simulink model "complete_model_sim_nolib"  (R2023b)
settings: Solver=VariableStepAuto  StartTime=0.0  StopTime=1e4  RelTol=1e-3
values from neighbouring files (symbols this model uses):
  a = 6.851221970532768e+03    (= 6851.22197053)    [complete_model.m]
  alpha1 = 0.4    [complete_model.m]
  alpha2 = 0.1    [complete_model.m]
  alpha3 = 0.5    [complete_model.m]
  D = zeros(3)    [complete_model.m]
  e = 0    [complete_model.m]
  FOV_earth = deg2rad(33)    [complete_model.m]
  FOV_sun = deg2rad(100)    [complete_model.m]
  freq_earth = 5    [complete_model.m]
  freq_mag = 5    [complete_model.m]
  freq_sun = 5    [complete_model.m]
  I = diag([I1 I2 I3])    [complete_model.m]    (also in compute_integral.m = I + (y(i + 1) + y(i) ) * (t(i + 1) - t(i)) * 0.5)
  Iinv = I\eye(3)    [complete_model.m]
  jb = [0.01; 0.05; 0.01]    [complete_model.m]
  k_gain = (4*pi/T) * (1 + sin(chsi)) * I2    [complete_model.m]
  mu = astroConstants(13)    [complete_model.m]
  n = sqrt(mu/a^3)    [complete_model.m]
  omega0 = 0.06 * rand(3,1)    [complete_model.m]
  omegaE = deg2rad(15)/3600    [complete_model.m]
  rs = -rr    [complete_model.m]
  s0 = 2*pi*rand(3,1)    [complete_model.m]
  tol = 0.2    [complete_model.m]
undefined symbols (not defined in the file or in its folder): gh, magnitude
libraries: cstextras x3, matrix_library x2, simulink_extras x1
(part 2 of 3)

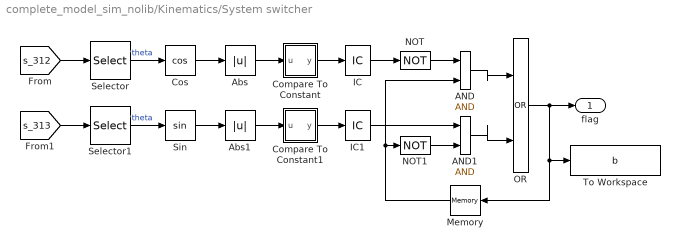
== system complete_model_sim_nolib/Kinematics/System switcher ==
  AND : Logic  IconShape=distinctive  AllPortsSameDT=off  OutDataTypeStr=boolean
  AND1 : Logic  IconShape=distinctive  AllPortsSameDT=off  OutDataTypeStr=boolean
  Abs : Abs  SaturateOnIntegerOverflow=off
  Abs1 : Abs  SaturateOnIntegerOverflow=off
  Compare To Constant : Subsystem  mask(Compare To Constant){relop=<, const=tol, OutDataTypeStr=boolean, ZeroCross=on}
      mask prompts: relop "Simulink:masks:Operator_MP"; const "Simulink:masks:ConstantValue_MP"; OutDataTypeStr "Simulink:masks:OutputDataType_MP"; ZeroCross "Simulink:masks:EnableZerocrossingDetection_MP"
      mask help: Simulink:masks:CompareToConstant_MD
      mask init: same as complete_model_sim_nolib/Control/De-Tumbling Bdot control1/Compare To Constant
      settings: LibrarySourceBlock=|
      | simulink/Logic and Bit
      | Operations/Compare
      | To Constant
      mask TypeOptions relop: == | ~= | < | <= | >= | >
      mask TypeOptions OutDataTypeStr: Simulink:masks:uint8 | Simulink:masks:boolean
      mask Callback ZeroCross: sl('zeroCrossEnable', gcbh);
      mask Display: disp(str)
  Compare To Constant1 : Subsystem  mask(Compare To Constant){relop=<, const=tol, OutDataTypeStr=boolean, ZeroCross=on}
      mask prompts: relop "Simulink:masks:Operator_MP"; const "Simulink:masks:ConstantValue_MP"; OutDataTypeStr "Simulink:masks:OutputDataType_MP"; ZeroCross "Simulink:masks:EnableZerocrossingDetection_MP"
      mask help: Simulink:masks:CompareToConstant_MD
      mask init: same as complete_model_sim_nolib/Control/De-Tumbling Bdot control1/Compare To Constant
      settings: LibrarySourceBlock=|
      | simulink/Logic and Bit
      | Operations/Compare
      | To Constant
      mask TypeOptions relop: == | ~= | < | <= | >= | >
      mask TypeOptions OutDataTypeStr: Simulink:masks:uint8 | Simulink:masks:boolean
      mask Callback ZeroCross: sl('zeroCrossEnable', gcbh);
      mask Display: disp(str)
  Cos : Trigonometry  Operator=cos
  IC : InitialCondition  Value=0
  IC1 : InitialCondition  Value=0
  Memory : Memory  InitialCondition=1
  NOT : Logic  Operator=NOT  IconShape=distinctive  AllPortsSameDT=off  OutDataTypeStr=boolean
  NOT1 : Logic  Operator=NOT  IconShape=distinctive  AllPortsSameDT=off  OutDataTypeStr=boolean
  OR : Logic  Operator=OR  IconShape=distinctive  AllPortsSameDT=off  OutDataTypeStr=boolean
  Selector : Selector  InputPortWidth=3  IndexOptions=Index vector (dialog)  Indices=2  OutputSizes=1
  Selector1 : Selector  InputPortWidth=3  IndexOptions=Index vector (dialog)  Indices=2  OutputSizes=1
  Sin : Trigonometry
  To Workspace : ToWorkspace  VariableName=b  SaveFormat=Timeseries  SampleTime=-1
  flag : Outport
  wires:
  Cos/1 -> Abs/1
  [s_312] -> Selector/1
  Compare To Constant/1(y) -> IC/1
  Selector1/1 -> Sin/1  "theta"
  Abs/1 -> Compare To Constant/1(u)
  Compare To Constant1/1(y) -> IC1/1
  Selector/1 -> Cos/1  "theta"
  Abs1/1 -> Compare To Constant1/1(u)
  Sin/1 -> Abs1/1
  [s_313] -> Selector1/1
  IC/1 -> NOT/1
  NOT/1 -> AND/1
  AND/1 -> OR/1
  NOT1/1 -> AND1/2
  IC1/1 -> AND1/1
  AND1/1 -> OR/2
  OR/1 -> To Workspace/1, Memory/1, flag/1
  Memory/1 -> AND/2, NOT1/1

== system complete_model_sim_nolib/Magnetometer/Band-Limited White Noise ==
  Output : Gain  Gain=sqrt(Cov)/sqrt(Ts(1))  SaturateOnIntegerOverflow=on  OutDataTypeStr=Inherit: Same as input  ParamDataTypeStr=Inherit: Same as input
  White Noise : RandomNumber  DisableCoverage=on  Seed=seed  SampleTime=Ts
  y : Outport
  wires:
  Output/1 -> y/1
  White Noise/1 -> Output/1

== system complete_model_sim_nolib/Magnetometer/Band-Limited White Noise1 ==
  Output : Gain  Gain=sqrt(Cov)/sqrt(Ts(1))  SaturateOnIntegerOverflow=on  OutDataTypeStr=Inherit: Same as input  ParamDataTypeStr=Inherit: Same as input
  White Noise : RandomNumber  DisableCoverage=on  Seed=seed  SampleTime=Ts
  y : Outport
  wires:
  Output/1 -> y/1
  White Noise/1 -> Output/1

== system complete_model_sim_nolib/Magnetometer/Band-Limited White Noise2 ==
  Output : Gain  Gain=sqrt(Cov)/sqrt(Ts(1))  SaturateOnIntegerOverflow=on  OutDataTypeStr=Inherit: Same as input  ParamDataTypeStr=Inherit: Same as input
  White Noise : RandomNumber  DisableCoverage=on  Seed=seed  SampleTime=Ts
  y : Outport
  wires:
  Output/1 -> y/1
  White Noise/1 -> Output/1

== system complete_model_sim_nolib/Magnetometer/Normalize Vector ==
  In1 : Inport
  Constant : Constant
  Demux : Demux  Outputs=[-1 1]
  Divide : Product  Inputs=*/  OutDataTypeStr=double
  Ground : Ground
  Math Function : Math  Operator=square  SignedPower=on
  Math Function1 : Math  Operator=sqrt  SignedPower=on
  Mux : Mux  Inputs=2
  Mux1 : Mux  Inputs=2
  Product : Product  RndMeth=Zero
  Sum of Elements : Sum  Inputs=+
  Switch : Switch  Criteria=u2 > Threshold  Threshold=maxzero  SaturateOnIntegerOverflow=off  InputSameDT=off
  Out1 : Outport  VectorParamsAs1DForOutWhenUnconnected=off
  wires:
  Ground/1 -> Product/2
  Product/1 -> Mux1/1
  Constant/1 -> Mux1/2
  Mux1/1 -> Switch/3
  Sum of Elements/1 -> Math Function1/1
  Math Function/1 -> Sum of Elements/1
  Demux/2 -> Divide/2
  Demux/1 -> Divide/1
  Switch/1 -> Demux/1
  Mux/1 -> Switch/1
  Math Function1/1 -> Mux/2, Switch/2
  In1/1 -> Product/1, Math Function/1, Mux/1
  Divide/1 -> Out1/1

== system complete_model_sim_nolib/Sun Sensor/FOV CHECK ==
  In1 : Inport
  Acos : Trigonometry  Operator=acos
  Dot Product : DotProduct  OutDataTypeStr=Inherit: Inherit via internal rule
  FOV angle : Constant  Value=FOV_sun
  Less Than : RelationalOperator  Operator=<  OutDataTypeStr=boolean  RndMeth=Simplest  InputSameDT=off
  optical axis : Constant  Value=[0;0;1]
  b : Outport
  wires:
  optical axis/1 -> Dot Product/1
  In1/1 -> Dot Product/2
  Dot Product/1 -> Acos/1
  FOV angle/1 -> Less Than/2
  Acos/1 -> Less Than/1
  Less Than/1 -> b/1

== system complete_model_sim_nolib/Sun Sensor/Sun Sensor Modeling ==
  Sb : Inport
  Cross Product : Subsystem  mask(CrossProduct){}
      mask help: Simulink:masks:MatLibCrossProduct_MD
      settings: LibrarySourceBlock=|
      | simulink/Matrix
      | Operations/Cross Product
      mask Display: disp('cross')
  Normalize Vector : Subsystem  mask(Normalize Vector){maxzero=0}
      mask prompts: maxzero "Maximum modulus to treat vector as zero:"
      mask help:
      | Normalize a vector.
      | Output is the unit vector parallel to the input vector. Input can be vector of any size.
      | If the modulus of the input is lower or equal than specified, the output is set to zeros(size(u)).
      settings: LibrarySourceBlock=vrlib/Utilities/Normalize Vector
      mask Help: helpview(vrmfunc('FnHelpTopic'), 'vr_normalizevector');
      mask Display: disp('Normalize')
  Normalize Vector1 : Subsystem  mask(Normalize Vector){maxzero=0}
      mask prompts: maxzero "Maximum modulus to treat vector as zero:"
      mask help:
      | Normalize a vector.
      | Output is the unit vector parallel to the input vector. Input can be vector of any size.
      | If the modulus of the input is lower or equal than specified, the output is set to zeros(size(u)).
      settings: LibrarySourceBlock=vrlib/Utilities/Normalize Vector
      mask Help: helpview(vrmfunc('FnHelpTopic'), 'vr_normalizevector');
      mask Display: disp('Normalize')
  Product : Product
  Random Number : RandomNumber  Variance=tan(deg2rad(1/60))^2*0.1  SampleTime=0.1
  Sum2 : Sum
  Uniform Random Number : UniformRandomNumber  SampleTime=1/freq_sun
  Uniform Random Number1 : UniformRandomNumber  SampleTime=1/freq_sun
  Uniform Random Number2 : UniformRandomNumber  SampleTime=1/freq_sun
  Vector Concatenate : Concatenate  NumInputs=3
  Zero-Order Hold : ZeroOrderHold  SampleTime=1/freq_sun
  s3 : Outport
  wires:
  Zero-Order Hold/1 -> Cross Product/2(b), Sum2/2  "Sb"
  Sum2/1 -> Normalize Vector/1(In1)  "q"
  Uniform Random Number1/1 -> Vector Concatenate/2
  Vector Concatenate/1 -> Cross Product/1(a)
  Uniform Random Number2/1 -> Vector Concatenate/3
  Normalize Vector/1(Out1) -> s3/1
  Uniform Random Number/1 -> Vector Concatenate/1
  Product/1 -> Sum2/1
  Random Number/1 -> Product/1
  Sb/1 -> Zero-Order Hold/1
  Cross Product/1(y) -> Normalize Vector1/1(In1)
  Normalize Vector1/1(Out1) -> Product/2

== system complete_model_sim_nolib/kep_dyn/r_norm ==
  e : Inport
  theta : Inport  Port=2
  Constant : Constant  Value=a
  Constant1 : Constant
  Cos : Trigonometry  Operator=cos
  Divide : Product  Inputs=*/
  Power : Math  Operator=magnitude^2
  Product : Product
  Product1 : Product
  Sum : Sum  Inputs=+-
  Sum2 : Sum
  r : Outport
  wires:
  e/1 -> Product1/2, Power/1
  Power/1 -> Sum/2
  Constant1/1 -> Sum2/2, Sum/1
  Sum/1 -> Product/2
  Constant/1 -> Product/1
  theta/1 -> Cos/1
  Cos/1 -> Product1/1
  Product1/1 -> Sum2/1
  Product/1 -> Divide/1
  Sum2/1 -> Divide/2
  Divide/1 -> r/1

== system complete_model_sim_nolib/kep_dyn/theta integration ==
  theta : Inport
  e : Inport  Port=2
  Constant : Constant  Value=n
  Constant2 : Constant
  Constant3 : Constant  Value=3/2
  Cos : Trigonometry  Operator=cos
  Divide : Product  Inputs=*/
  Math Function : Math  Operator=square
  Math Function1 : Math  Operator=square
  Math Function2 : Math  Operator=pow
  Product : Product
  Product1 : Product
  Sum : Sum
  Sum1 : Sum  Inputs=+-
  theta_dot : Outport
  wires:
  Product1/1 -> Divide/1
  Product/1 -> Sum/2
  Math Function2/1 -> Divide/2
  Sum1/1 -> Math Function2/1
  Constant2/1 -> Sum1/1, Sum/1
  Math Function1/1 -> Sum1/2
  e/1 -> Product/2, Math Function1/1
  Constant3/1 -> Math Function2/2
  Constant/1 -> Product1/1
  Sum/1 -> Math Function/1
  Math Function/1 -> Product1/2
  Cos/1 -> Product/1
  theta/1 -> Cos/1
  Divide/1 -> theta_dot/1

== system complete_model_sim_nolib/relative kinematics/Subsystem ==
  theta : Inport
  Constant3 : Constant
  Constant4 : Constant  Value=0
  Cos2 : Trigonometry  Operator=cos
  Cos3 : Trigonometry
  Gain : Gain  Gain=-1
  Matrix Concatenate1 : Concatenate  NumInputs=3  Mode=Multidimensional array  ConcatenateDimension=2
  Vector Concatenate : Concatenate  NumInputs=3
  Vector Concatenate1 : Concatenate  NumInputs=3
  Vector Concatenate2 : Concatenate  NumInputs=3
  A_PL : Outport
  wires:
  Constant4/1 -> Vector Concatenate2/2, Vector Concatenate/3, Vector Concatenate1/3, Vector Concatenate2/1
  Vector Concatenate/1 -> Matrix Concatenate1/1
  Cos2/1 -> Vector Concatenate1/2, Vector Concatenate/1
  Gain/1 -> Vector Concatenate1/1
  Cos3/1 -> Vector Concatenate/2, Gain/1
  Constant3/1 -> Vector Concatenate2/3
  Vector Concatenate2/1 -> Matrix Concatenate1/3
  Vector Concatenate1/1 -> Matrix Concatenate1/2
  theta/1 -> Cos2/1, Cos3/1
  Matrix Concatenate1/1 -> A_PL/1  "A_PL"

== system complete_model_sim_nolib/Attitude Determination  1/Enabled Subsystem/S ==
  q : Inport
  p : Inport  Port=2
  Cross Product : Subsystem  mask(CrossProduct){}
      mask help: Simulink:masks:MatLibCrossProduct_MD
      settings: LibrarySourceBlock=|
      | simulink/Matrix
      | Operations/Cross Product
      mask Display: disp('cross')
  Cross Product1 : Subsystem  mask(CrossProduct){}
      mask help: Simulink:masks:MatLibCrossProduct_MD
      settings: LibrarySourceBlock=|
      | simulink/Matrix
      | Operations/Cross Product
      mask Display: disp('cross')
  Matrix Concatenate : Concatenate  NumInputs=3  Mode=Multidimensional array  ConcatenateDimension=2
  Normalize Vector : Subsystem  mask(Normalize Vector){maxzero=0}
      mask prompts: maxzero "Maximum modulus to treat vector as zero:"
      mask help:
      | Normalize a vector.
      | Output is the unit vector parallel to the input vector. Input can be vector of any size.
      | If the modulus of the input is lower or equal than specified, the output is set to zeros(size(u)).
      settings: LibrarySourceBlock=vrlib/Utilities/Normalize Vector
      mask Help: helpview(vrmfunc('FnHelpTopic'), 'vr_normalizevector');
      mask Display: disp('Normalize')
  S : Outport
  wires:
  p/1 -> Matrix Concatenate/1, Cross Product/1(a), Cross Product1/1(a)
  q/1 -> Cross Product/2(b)
  Normalize Vector/1(Out1) -> Matrix Concatenate/2, Cross Product1/2(b)
  Matrix Concatenate/1 -> S/1
  Cross Product1/1(y) -> Matrix Concatenate/3
  Cross Product/1(y) -> Normalize Vector/1(In1)

== system complete_model_sim_nolib/Attitude Determination  1/Enabled Subsystem/V ==
  b : Inport
  a : Inport  Port=2
  Cross Product : Subsystem  mask(CrossProduct){}
      mask help: Simulink:masks:MatLibCrossProduct_MD
      settings: LibrarySourceBlock=|
      | simulink/Matrix
      | Operations/Cross Product
      mask Display: disp('cross')
  Cross Product1 : Subsystem  mask(CrossProduct){}
      mask help: Simulink:masks:MatLibCrossProduct_MD
      settings: LibrarySourceBlock=|
      | simulink/Matrix
      | Operations/Cross Product
      mask Display: disp('cross')
  Matrix Concatenate : Concatenate  NumInputs=3  Mode=Multidimensional array  ConcatenateDimension=2
  Normalize Vector : Subsystem  mask(Normalize Vector){maxzero=0}
      mask prompts: maxzero "Maximum modulus to treat vector as zero:"
      mask help:
      | Normalize a vector.
      | Output is the unit vector parallel to the input vector. Input can be vector of any size.
      | If the modulus of the input is lower or equal than specified, the output is set to zeros(size(u)).
      settings: LibrarySourceBlock=vrlib/Utilities/Normalize Vector
      mask Help: helpview(vrmfunc('FnHelpTopic'), 'vr_normalizevector');
      mask Display: disp('Normalize')
  V : Outport
  wires:
  Cross Product1/1(y) -> Matrix Concatenate/3
  Matrix Concatenate/1 -> V/1
  Normalize Vector/1(Out1) -> Cross Product1/2(b), Matrix Concatenate/2
  Cross Product/1(y) -> Normalize Vector/1(In1)
  b/1 -> Cross Product/2(b)
  a/1 -> Cross Product1/1(a), Cross Product/1(a), Matrix Concatenate/1

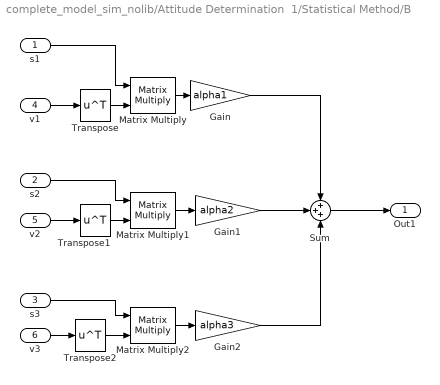
== system complete_model_sim_nolib/Attitude Determination  1/Statistical Method/B ==
  s1 : Inport
  s2 : Inport  Port=2
  s3 : Inport  Port=3
  v1 : Inport  Port=4
  v2 : Inport  Port=5
  v3 : Inport  Port=6
  Gain : Gain  Gain=alpha1
  Gain1 : Gain  Gain=alpha2
  Gain2 : Gain  Gain=alpha3
  Matrix Multiply : Product  Multiplication=Matrix(*)
  Matrix Multiply1 : Product  Multiplication=Matrix(*)
  Matrix Multiply2 : Product  Multiplication=Matrix(*)
  Sum : Sum  Inputs=+++
  Transpose : Math  Operator=transpose
  Transpose1 : Math  Operator=transpose
  Transpose2 : Math  Operator=transpose
  Out1 : Outport
  wires:
  v1/1 -> Transpose/1
  Transpose/1 -> Matrix Multiply/2
  s1/1 -> Matrix Multiply/1
  Transpose1/1 -> Matrix Multiply1/2
  s2/1 -> Matrix Multiply1/1
  Transpose2/1 -> Matrix Multiply2/2
  v3/1 -> Transpose2/1
  Sum/1 -> Out1/1
  Matrix Multiply/1 -> Gain/1
  Matrix Multiply1/1 -> Gain1/1
  Matrix Multiply2/1 -> Gain2/1
  Gain/1 -> Sum/1
  Gain1/1 -> Sum/2
  Gain2/1 -> Sum/3
  v2/1 -> Transpose1/1
  s3/1 -> Matrix Multiply2/1

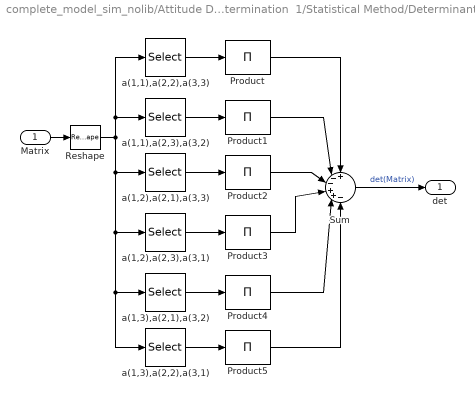
== system complete_model_sim_nolib/Attitude Determination  1/Statistical Method/Determinant of 3x3 Matrix ==
  Matrix : Inport  PortDimensions=[3 3]
  Product{,1..5} (6 alike) : Product  Inputs=1  SaturateOnIntegerOverflow=on  OutDataTypeStr=Inherit: Same as first input
  Reshape : Reshape  OutputDimensionality=Column vector (2-D)
  Sum : Sum  Inputs=+--++-  SaturateOnIntegerOverflow=on
  a(1,1),a(2,2),a(3,3) : Selector  InputPortWidth=9  IndexOptions=Index vector (dialog)  Indices=[1 5 9]  OutputSizes=1
  a(1,1),a(2,3),a(3,2) : Selector  InputPortWidth=9  IndexOptions=Index vector (dialog)  Indices=[1 6 8]  OutputSizes=1
  a(1,2),a(2,1),a(3,3) : Selector  InputPortWidth=9  IndexOptions=Index vector (dialog)  Indices=[2 4 9]  OutputSizes=1
  a(1,2),a(2,3),a(3,1) : Selector  InputPortWidth=9  IndexOptions=Index vector (dialog)  Indices=[3 4 8]  OutputSizes=1
  a(1,3),a(2,1),a(3,2) : Selector  InputPortWidth=9  IndexOptions=Index vector (dialog)  Indices=[2 6 7]  OutputSizes=1
  a(1,3),a(2,2),a(3,1) : Selector  InputPortWidth=9  IndexOptions=Index vector (dialog)  Indices=[3 5 7]  OutputSizes=1
  det : Outport  PortDimensions=1  VectorParamsAs1DForOutWhenUnconnected=off
  wires:
  Reshape/1 -> a(1,1),a(2,3),a(3,2)/1, a(1,1),a(2,2),a(3,3)/1, a(1,3),a(2,2),a(3,1)/1, a(1,3),a(2,1),a(3,2)/1, a(1,2),a(2,3),a(3,1)/1, a(1,2),a(2,1),a(3,3)/1
  Sum/1 -> det/1  "det(Matrix)"
  Matrix/1 -> Reshape/1
  Product5/1 -> Sum/6
  Product4/1 -> Sum/5
  Product3/1 -> Sum/4
  Product2/1 -> Sum/3
  Product1/1 -> Sum/2
  Product/1 -> Sum/1
  a(1,3),a(2,2),a(3,1)/1 -> Product5/1
  a(1,3),a(2,1),a(3,2)/1 -> Product4/1
  a(1,2),a(2,3),a(3,1)/1 -> Product3/1
  a(1,2),a(2,1),a(3,3)/1 -> Product2/1
  a(1,1),a(2,3),a(3,2)/1 -> Product1/1
  a(1,1),a(2,2),a(3,3)/1 -> Product/1

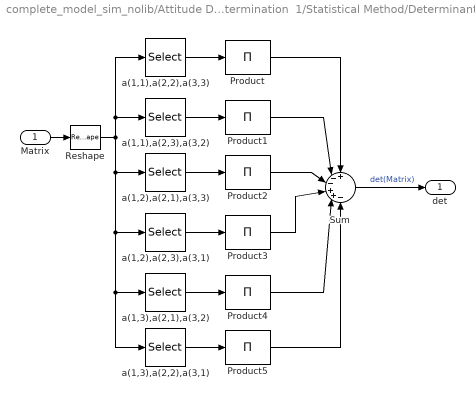
== system complete_model_sim_nolib/Attitude Determination  1/Statistical Method/Determinant of 3x3 Matrix1 ==
  Matrix : Inport  PortDimensions=[3 3]
  Product{,1..5} (6 alike) : Product  Inputs=1  SaturateOnIntegerOverflow=on  OutDataTypeStr=Inherit: Same as first input
  Reshape : Reshape  OutputDimensionality=Column vector (2-D)
  Sum : Sum  Inputs=+--++-  SaturateOnIntegerOverflow=on
  a(1,1),a(2,2),a(3,3) : Selector  InputPortWidth=9  IndexOptions=Index vector (dialog)  Indices=[1 5 9]  OutputSizes=1
  a(1,1),a(2,3),a(3,2) : Selector  InputPortWidth=9  IndexOptions=Index vector (dialog)  Indices=[1 6 8]  OutputSizes=1
  a(1,2),a(2,1),a(3,3) : Selector  InputPortWidth=9  IndexOptions=Index vector (dialog)  Indices=[2 4 9]  OutputSizes=1
  a(1,2),a(2,3),a(3,1) : Selector  InputPortWidth=9  IndexOptions=Index vector (dialog)  Indices=[3 4 8]  OutputSizes=1
  a(1,3),a(2,1),a(3,2) : Selector  InputPortWidth=9  IndexOptions=Index vector (dialog)  Indices=[2 6 7]  OutputSizes=1
  a(1,3),a(2,2),a(3,1) : Selector  InputPortWidth=9  IndexOptions=Index vector (dialog)  Indices=[3 5 7]  OutputSizes=1
  det : Outport  PortDimensions=1  VectorParamsAs1DForOutWhenUnconnected=off
  wires:
  a(1,1),a(2,2),a(3,3)/1 -> Product/1
  a(1,1),a(2,3),a(3,2)/1 -> Product1/1
  a(1,2),a(2,1),a(3,3)/1 -> Product2/1
  a(1,2),a(2,3),a(3,1)/1 -> Product3/1
  a(1,3),a(2,1),a(3,2)/1 -> Product4/1
  a(1,3),a(2,2),a(3,1)/1 -> Product5/1
  Product/1 -> Sum/1
  Product1/1 -> Sum/2
  Product2/1 -> Sum/3
  Product3/1 -> Sum/4
  Product4/1 -> Sum/5
  Product5/1 -> Sum/6
  Matrix/1 -> Reshape/1
  Sum/1 -> det/1  "det(Matrix)"
  Reshape/1 -> a(1,2),a(2,1),a(3,3)/1, a(1,2),a(2,3),a(3,1)/1, a(1,3),a(2,1),a(3,2)/1, a(1,3),a(2,2),a(3,1)/1, a(1,1),a(2,2),a(3,3)/1, a(1,1),a(2,3),a(3,2)/1

== system complete_model_sim_nolib/Control/De-Tumbling Bdot control1/Compare To Constant ==
  u : Inport
  Compare : RelationalOperator  OutDataTypeStr=boolean
  Constant : Constant  DisableCoverage=on  Value=const  OutDataTypeStr=Inherit: Inherit via back propagation
  y : Outport
  wires:
  u/1 -> Compare/1
  Constant/1 -> Compare/2
  Compare/1 -> y/1

== system complete_model_sim_nolib/Control/De-Tumbling Bdot control1/Compare To Constant1 ==
  u : Inport
  Compare : RelationalOperator  Operator=<=  OutDataTypeStr=boolean
  Constant : Constant  DisableCoverage=on  Value=const  OutDataTypeStr=Inherit: Inherit via back propagation
  y : Outport
  wires:
  u/1 -> Compare/1
  Constant/1 -> Compare/2
  Compare/1 -> y/1

== system complete_model_sim_nolib/Control/De-Tumbling Bdot control1/Discrete Derivative1 ==
  note: ( U(k) - U(k-1) )
  note: U(k)
  U : Inport
  Data Type Duplicate : DataTypeDuplicate  DisableCoverage=on  NumInputPorts=3
  Diff : Sum  Description=Add in CPU  Inputs=+-  OutMin=OutMin  OutMax=OutMax  OutDataTypeStr=diffDT
  TSamp : SampleTimeMath  DisableCoverage=on  TsampMathOp=/  weightValue=inverseGainval  TsampMathImp=Offline Scaling Adjustment
  UD : UnitDelay  Description=Store in Global RAM  DisableCoverage=on  InitialCondition=ICPrevScaledInput  SampleTime=-1  HasFrameUpgradeWarning=on
  Y : Outport  OutMin=OutMin  OutMax=OutMax  InitialOutput=0
  wires:
  U/1 -> TSamp/1
  UD/1 -> Diff/2, Data Type Duplicate/3  "U(k-1)"
  Diff/1 -> Y/1, Data Type Duplicate/1
  TSamp/1 -> UD/1, Diff/1, Data Type Duplicate/2

== system complete_model_sim_nolib/Control/De-Tumbling Bdot control1/Discrete Varying Lowpass1 ==
  u : Inport
  frequency : Inport  Port=2
  FOS : cstextras/DiscreteFirstOrderSection  VariantControl=(default)  Ts=Ts  w0=w0
  y : Outport  VectorParamsAs1DForOutWhenUnconnected=off
  wires:
  u/1 -> FOS/1
  frequency/1 -> FOS/2
  FOS/1 -> y/1

== system complete_model_sim_nolib/Control/De-Tumbling Bdot control1/Normalize Vector ==
  In1 : Inport
  Constant : Constant
  Demux : Demux  Outputs=[-1 1]
  Divide : Product  Inputs=*/  OutDataTypeStr=double
  Ground : Ground
  Math Function : Math  Operator=square  SignedPower=on
  Math Function1 : Math  Operator=sqrt  SignedPower=on
  Mux : Mux  Inputs=2
  Mux1 : Mux  Inputs=2
  Product : Product  RndMeth=Zero
  Sum of Elements : Sum  Inputs=+
  Switch : Switch  Criteria=u2 > Threshold  Threshold=maxzero  SaturateOnIntegerOverflow=off  InputSameDT=off
  Out1 : Outport  VectorParamsAs1DForOutWhenUnconnected=off
  wires:
  Ground/1 -> Product/2
  Product/1 -> Mux1/1
  Constant/1 -> Mux1/2
  Mux1/1 -> Switch/3
  Sum of Elements/1 -> Math Function1/1
  Math Function/1 -> Sum of Elements/1
  Demux/2 -> Divide/2
  Demux/1 -> Divide/1
  Switch/1 -> Demux/1
  Mux/1 -> Switch/1
  Math Function1/1 -> Mux/2, Switch/2
  In1/1 -> Product/1, Math Function/1, Mux/1
  Divide/1 -> Out1/1

== system complete_model_sim_nolib/Control/Slew Maneuver/Control Logic ==
  u : Inport
  B_m : Inport  Port=2
  Abs1 : Abs  SaturateOnIntegerOverflow=off
  Compare To Constant : Subsystem  mask(Compare To Constant){relop=>, const=1e-5, OutDataTypeStr=boolean, ZeroCross=on}
      mask prompts: relop "Simulink:masks:Operator_MP"; const "Simulink:masks:ConstantValue_MP"; OutDataTypeStr "Simulink:masks:OutputDataType_MP"; ZeroCross "Simulink:masks:EnableZerocrossingDetection_MP"
      mask help: Simulink:masks:CompareToConstant_MD
      mask init: same as complete_model_sim_nolib/Control/De-Tumbling Bdot control1/Compare To Constant
      settings: LibrarySourceBlock=|
      | simulink/Logic and Bit
      | Operations/Compare
      | To Constant
      mask TypeOptions relop: == | ~= | < | <= | >= | >
      mask TypeOptions OutDataTypeStr: Simulink:masks:uint8 | Simulink:masks:boolean
      mask Callback ZeroCross: sl('zeroCrossEnable', gcbh);
      mask Display: disp(str)
  Merge1 : Merge
  NOT : Logic  Operator=NOT  IconShape=distinctive  AllPortsSameDT=off  OutDataTypeStr=boolean
  Selector1 : Selector  InputPortWidth=3  IndexOptions=Index vector (dialog)  Indices=1  OutputSizes=1
  Subsystem : Subsystem
  Subsystem1 : Subsystem
  cmd : Outport
  wires:
  Abs1/1 -> Compare To Constant/1(u)
  Selector1/1 -> Abs1/1
  NOT/1 -> Subsystem/Enable
  Subsystem1/1(Out1) -> Merge1/1
  Compare To Constant/1(y) -> NOT/1, Subsystem1/Enable
  Subsystem/1(Out1) -> Merge1/2
  B_m/1 -> Selector1/1, Subsystem/1(Bm), Subsystem1/1(B_m)
  u/1 -> Subsystem/2(u), Subsystem1/2(u)
  Merge1/1 -> cmd/1

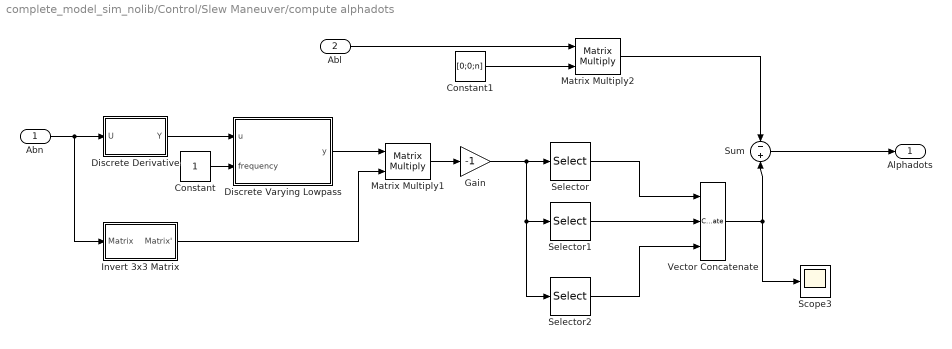
== system complete_model_sim_nolib/Control/Slew Maneuver/compute alphadots ==
  Abn : Inport
  Abl : Inport  Port=2
  Constant : Constant
  Constant1 : Constant  Value=[0;0;n]
  Discrete Derivative : Subsystem  mask(Discrete Derivative){gainval=1.0, ICPrevScaledInput=0.0, InputProcessing=Elements as channels (sample based), OutMin=[], OutMax=[], OutDataTypeStr=Inherit: Inherit via internal rule, OutputDataTypeScalingMode=Inherit via internal rule, OutDataType=fixdt(1, 16), OutScaling=2^-10, LockScale=off, RndMeth=Floor, DoSatur=off}
      mask prompts: gainval "Simulink:masks:GainValue_MP"; ICPrevScaledInput "Simulink:masks:InitialConditionForPreviousWeightedInputKuTs_MP"; InputProcessing "Simulink:masks:InputProcessing_MP"; OutMin "Simulink:masks:OutputMinimum_MP"; OutMax "Simulink:masks:OutputMaximum_MP"; OutDataTypeStr "Simulink:masks:OutputDataType_MP"; OutputDataTypeScalingMode "Simulink:masks:OutputDataTypeMode_MP"; OutDataType "Simulink:masks:OutputDataTypeegFixdt116Fixdtsingle_MP"; OutScaling "Simulink:masks:OutputScalingSlopeEg29OrSlopeBias_MP"; LockScale "Simulink:masks:LockOutputDataTypeAgainstFxpTools_MP"; RndMeth "Simulink:masks:IntegerRoundingMode_MP"; DoSatur "Simulink:masks:SaturateToMaxOrMinWhenOverflowsOccur_MP"
      mask help: Simulink:masks:DiscreteDerivative_MD
      mask init: same as complete_model_sim_nolib/Control/De-Tumbling Bdot control1/Discrete Derivative1
      settings: LibrarySourceBlock=simulink/Discrete/Discrete Derivative
      mask TypeOptions InputProcessing: Simulink:masks:ColumnsAsChannelsFrameBased | Simulink:masks:ElementsAsChannelsSampleBased
      mask Callback OutDataTypeStr: fixptdialog(gcbh)
      mask TypeOptions OutputDataTypeScalingMode: double | single | int8 | uint8 | int16 | uint16 | int32 | uint32 | Specify via dialog | Inherit via internal rule | Inherit via back propagation
      mask Callback OutputDataTypeScalingMode: fixptdialog(gcbh)
      mask Callback OutDataType: fixptdialog(gcbh)
      mask TypeOptions RndMeth: Simulink:masks:Ceiling | Simulink:masks:Convergent | Simulink:masks:Floor | Simulink:masks:Nearest | Simulink:masks:Round | Simulink:masks:Simplest | Simulink:masks:Zero
      mask Display: text(0.5, 0.5, 'K (z-1)', 'horizontalAlignment', 'center', 'verticalAlignment', 'bottom');text(0.5, 0.5, 'Ts z', 'horizontalAlignment', 'center', 'verticalAlignment', 'top');plot([0.3 0.7],[0.5 0.5]);
  Discrete Varying Lowpass : Subsystem  mask(Discrete Varying Lowpass){N=1, w0=0, Ts=1/30}
      mask prompts: N "Control:simulink:VaryingLowpassLabel1"; w0 "Control:simulink:VaryingLowpassLabel2"; Ts "Control:simulink:VaryingLowpassLabel3"
      mask help: Control:simulink:VaryingLowpass2
      mask init: same as complete_model_sim_nolib/ Actuators/Discrete Varying Lowpass
      settings: LibrarySourceBlock=cstblocks/Linear Parameter Varying/Discrete Varying Lowpass
      mask Help: eval('helpview(''control'',''VaryingLowpassDT'');')
      mask DialogControl N Prompt: Filter order:
      mask DialogControl w0 Prompt: Pre-warping frequency w0 (rad/s):
      mask DialogControl Ts Prompt: Sample time Ts:
      mask Display:
      | image('lowpass_dt.png',[0.1 0 0.8 1]);
      | port_label('input', 2, 'freq');
  Gain : Gain  Gain=-1
  Invert 3x3 Matrix : Subsystem
      settings: LibrarySourceBlock=|
      | aerolibutil/Invert
      | 3x3 Matrix
  Matrix Multiply1 : Product  Multiplication=Matrix(*)
  Matrix Multiply2 : Product  Multiplication=Matrix(*)
  Scope3 : Scope
  Selector : Selector  NumberOfDimensions=2  InputPortWidth=3  IndexOptions=Index vector (dialog),Index vector (dialog)  Indices=3,2  OutputSizes=1,1
  Selector1 : Selector  NumberOfDimensions=2  InputPortWidth=3  IndexOptions=Index vector (dialog),Index vector (dialog)  Indices=1,3  OutputSizes=1,1
  Selector2 : Selector  NumberOfDimensions=2  InputPortWidth=3  IndexOptions=Index vector (dialog),Index vector (dialog)  Indices=2,1  OutputSizes=1,1
  Sum : Sum  Inputs=-+
  Vector Concatenate : Concatenate  NumInputs=3
  Alphadots : Outport
  wires:
  Selector/1 -> Vector Concatenate/1
  Matrix Multiply2/1 -> Sum/1
  Discrete Varying Lowpass/1(y) -> Matrix Multiply1/1
  Matrix Multiply1/1 -> Gain/1
  Constant1/1 -> Matrix Multiply2/2
  Abn/1 -> Invert 3x3 Matrix/1(Matrix), Discrete Derivative/1(U)
  Invert 3x3 Matrix/1(Matrix') -> Matrix Multiply1/2
  Gain/1 -> Selector2/1, Selector1/1, Selector/1
  Constant/1 -> Discrete Varying Lowpass/2(frequency)
  Sum/1 -> Alphadots/1
  Selector2/1 -> Vector Concatenate/3
  Selector1/1 -> Vector Concatenate/2
  Discrete Derivative/1(Y) -> Discrete Varying Lowpass/1(u)
  Vector Concatenate/1 -> Sum/2, Scope3/1
  Abl/1 -> Matrix Multiply2/1

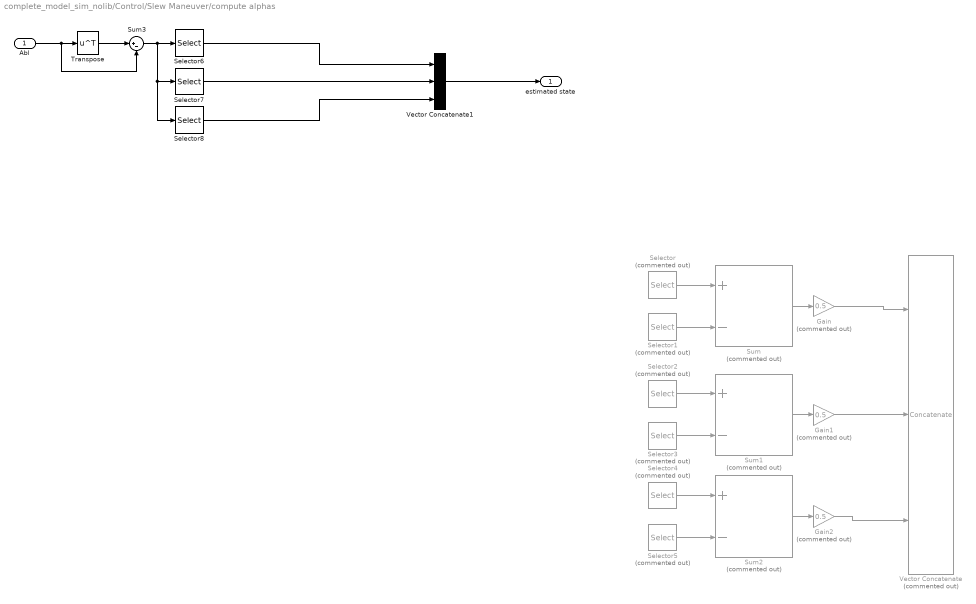
== system complete_model_sim_nolib/Control/Slew Maneuver/compute alphas ==
  Abl : Inport
  Gain : Gain  Commented=on  Gain=0.5
  Gain1 : Gain  Commented=on  Gain=0.5
  Gain2 : Gain  Commented=on  Gain=0.5
  Selector : Selector  Commented=on  NumberOfDimensions=2  InputPortWidth=3  IndexOptions=Index vector (dialog),Index vector (dialog)  Indices=2,3  OutputSizes=1,1
  Selector1 : Selector  Commented=on  NumberOfDimensions=2  InputPortWidth=3  IndexOptions=Index vector (dialog),Index vector (dialog)  Indices=3,2  OutputSizes=1,1
  Selector2 : Selector  Commented=on  NumberOfDimensions=2  InputPortWidth=3  IndexOptions=Index vector (dialog),Index vector (dialog)  Indices=3,1  OutputSizes=1,1
  Selector3 : Selector  Commented=on  NumberOfDimensions=2  InputPortWidth=3  IndexOptions=Index vector (dialog),Index vector (dialog)  Indices=1,3  OutputSizes=1,1
  Selector4 : Selector  Commented=on  NumberOfDimensions=2  InputPortWidth=3  IndexOptions=Index vector (dialog),Index vector (dialog)  Indices=1,2  OutputSizes=1,1
  Selector5 : Selector  Commented=on  NumberOfDimensions=2  InputPortWidth=3  IndexOptions=Index vector (dialog),Index vector (dialog)  Indices=2,1  OutputSizes=1,1
  Selector6 : Selector  NumberOfDimensions=2  InputPortWidth=3  IndexOptions=Index vector (dialog),Index vector (dialog)  Indices=3,2  OutputSizes=1,1
  Selector7 : Selector  NumberOfDimensions=2  InputPortWidth=3  IndexOptions=Index vector (dialog),Index vector (dialog)  Indices=1,3  OutputSizes=1,1
  Selector8 : Selector  NumberOfDimensions=2  InputPortWidth=3  IndexOptions=Index vector (dialog),Index vector (dialog)  Indices=2,1  OutputSizes=1,1
  Sum : Sum  Commented=on  Inputs=+-
  Sum1 : Sum  Commented=on  Inputs=+-
  Sum2 : Sum  Commented=on  Inputs=+-
  Sum3 : Sum  Inputs=|+-
  Transpose : Math  Operator=transpose
  Vector Concatenate : Concatenate  Commented=on  NumInputs=3
  Vector Concatenate1 : Concatenate  NumInputs=3
  estimated state : Outport
  wires:
  Selector1/1 -> Sum/2
  Selector/1 -> Sum/1
  Sum/1 -> Gain/1
  Selector2/1 -> Sum1/1
  Selector3/1 -> Sum1/2
  Selector4/1 -> Sum2/1
  Selector5/1 -> Sum2/2
  Sum1/1 -> Gain1/1
  Sum2/1 -> Gain2/1
  Gain/1 -> Vector Concatenate/1
  Gain1/1 -> Vector Concatenate/2
  Gain2/1 -> Vector Concatenate/3
  Abl/1 -> Sum3/2, Transpose/1
  Transpose/1 -> Sum3/1
  Sum3/1 -> Selector8/1, Selector7/1, Selector6/1
  Vector Concatenate1/1 -> estimated state/1
  Selector7/1 -> Vector Concatenate1/2
  Selector6/1 -> Vector Concatenate1/1
  Selector8/1 -> Vector Concatenate1/3

== system complete_model_sim_nolib/Disturbances/Magnetic Torque /compute Bn ==
  rN : Inport
  Cartesian to Spherical : simulink_extras/Transformations/Cartesian to Spherical
  Constant : Constant  Value=gh
  Demux : Demux  Outputs=3
  MATLAB Function : MATLAB Function  TreatAsAtomicUnit=on
  Matrix Multiply : Product  Multiplication=Matrix(*)
  Matrix Multiply1 : Product  Multiplication=Matrix(*)
  Subsystem : Subsystem
  Transpose : Math  Operator=transpose
  Bn : Outport
  wires:
  Subsystem/1(R_EN) -> Matrix Multiply/1, Transpose/1
  rN/1 -> Matrix Multiply/2
  Demux/1 -> Cartesian to Spherical/1
  Demux/2 -> Cartesian to Spherical/2
  Demux/3 -> Cartesian to Spherical/3
  Matrix Multiply/1 -> Demux/1
  Cartesian to Spherical/1 -> MATLAB Function/1(r)
  Cartesian to Spherical/2 -> MATLAB Function/2(theta)
  Cartesian to Spherical/3 -> MATLAB Function/3(phi)
  Transpose/1 -> Matrix Multiply1/1
  MATLAB Function/1(B) -> Matrix Multiply1/2
  Matrix Multiply1/1 -> Bn/1
  Constant/1 -> MATLAB Function/4(gh)

== system complete_model_sim_nolib/Horizon Sensor/EH sensor modeling/Cross Product ==
  note: Cross product of two 3x1 vectors a=[a1 a2 a3], b=[b1 b2 b3]:
      | y = a x b = (a2b3-a3b2)i + (a3b1-a1b3)j + (a1b2-a2b1)k
  a : Inport
  b : Inport  Port=2
  Element Product : Product  RndMeth=Simplest
  Selector2 : Selector  InputPortWidth=6  IndexOptions=Index vector (dialog)  Indices=[1 2 3]  OutputSizes=1
  Selector3 : Selector  InputPortWidth=6  IndexOptions=Index vector (dialog)  Indices=[4 5 6]  OutputSizes=1
  Sum : Sum  Inputs=+|-  RndMeth=Simplest
  a elements : Selector  InputPortWidth=3  IndexOptions=Index vector (dialog)  Indices=[2 3 1 3 1 2]  OutputSizes=1
  b elements : Selector  InputPortWidth=3  IndexOptions=Index vector (dialog)  Indices=[3 1 2 2 3 1]  OutputSizes=1
  y : Outport
  wires:
  Selector3/1 -> Sum/2
  Selector2/1 -> Sum/1
  Element Product/1 -> Selector2/1, Selector3/1
  b/1 -> b elements/1
  b elements/1 -> Element Product/2
  a elements/1 -> Element Product/1
  Sum/1 -> y/1
  a/1 -> a elements/1

== system complete_model_sim_nolib/Horizon Sensor/EH sensor modeling/Normalize Vector ==
  In1 : Inport
  Constant : Constant
  Demux : Demux  Outputs=[-1 1]
  Divide : Product  Inputs=*/  OutDataTypeStr=double
  Ground : Ground
  Math Function : Math  Operator=square  SignedPower=on
  Math Function1 : Math  Operator=sqrt  SignedPower=on
  Mux : Mux  Inputs=2
  Mux1 : Mux  Inputs=2
  Product : Product  RndMeth=Zero
  Sum of Elements : Sum  Inputs=+
  Switch : Switch  Criteria=u2 > Threshold  Threshold=maxzero  SaturateOnIntegerOverflow=off  InputSameDT=off
  Out1 : Outport  VectorParamsAs1DForOutWhenUnconnected=off
  wires:
  Ground/1 -> Product/2
  Product/1 -> Mux1/1
  Constant/1 -> Mux1/2
  Mux1/1 -> Switch/3
  Sum of Elements/1 -> Math Function1/1
  Math Function/1 -> Sum of Elements/1
  Demux/2 -> Divide/2
  Demux/1 -> Divide/1
  Switch/1 -> Demux/1
  Mux/1 -> Switch/1
  Math Function1/1 -> Mux/2, Switch/2
  In1/1 -> Product/1, Math Function/1, Mux/1
  Divide/1 -> Out1/1

== system complete_model_sim_nolib/Kinematics/Kinematics 312/A - s_312 ==
  A : Inport
  Asin : Trigonometry  Operator=asin
  Atan1 : Trigonometry  Operator=atan2
  Atan2 : Trigonometry  Operator=atan2
  Gain : Gain  Gain=-1
  Gain1 : Gain  Gain=-1
  Mux : Mux  Inputs=3
  Selector : Selector  NumberOfDimensions=2  InputPortWidth=3  IndexOptions=Index vector (dialog),Index vector (dialog)  Indices=2,1  OutputSizes=1,1
  Selector1 : Selector  NumberOfDimensions=2  InputPortWidth=3  IndexOptions=Index vector (dialog),Index vector (dialog)  Indices=2,2  OutputSizes=1,1
  Selector2 : Selector  NumberOfDimensions=2  InputPortWidth=3  IndexOptions=Index vector (dialog),Index vector (dialog)  Indices=2,3  OutputSizes=1,1
  Selector3 : Selector  NumberOfDimensions=2  InputPortWidth=3  IndexOptions=Index vector (dialog),Index vector (dialog)  Indices=1,3  OutputSizes=1,1
  Selector4 : Selector  NumberOfDimensions=2  InputPortWidth=3  IndexOptions=Index vector (dialog),Index vector (dialog)  Indices=3,3  OutputSizes=1,1
  s : Outport
  wires:
  Mux/1 -> s/1
  Selector4/1 -> Atan1/2  "a33"
  Atan1/1 -> Mux/3  "psi"
  Atan2/1 -> Mux/1  "phi"
  A/1 -> Selector2/1, Selector1/1, Selector/1, Selector3/1, Selector4/1
  Selector2/1 -> Asin/1  "a23"
  Selector3/1 -> Gain1/1  "a13"
  Selector1/1 -> Atan2/2  "a22"
  Selector/1 -> Gain/1  "a21"
  Asin/1 -> Mux/2  "theta"
  Gain/1 -> Atan2/1
  Gain1/1 -> Atan1/1

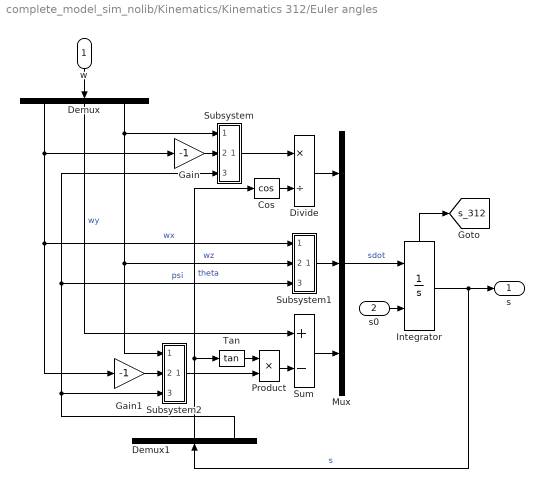
== system complete_model_sim_nolib/Kinematics/Kinematics 312/Euler angles ==
  w : Inport
  s0 : Inport  Port=2
  Cos : Trigonometry  Operator=cos
  Demux : Demux  Outputs=3
  Demux1 : Demux  Outputs=3
  Divide : Product  Inputs=*/
  Gain : Gain  Gain=-1
  Gain1 : Gain  Gain=-1
  Integrator : Integrator  InitialConditionSource=external  InitialCondition=s0  WrapState=on  WrappedStateUpperValue=2*pi  WrappedStateLowerValue=0  ShowStatePort=on
  Mux : Mux  Inputs=3
  Product : Product
  Subsystem : Subsystem
  Subsystem1 : Subsystem
  Subsystem2 : Subsystem
  Sum : Sum  Inputs=+-
  Tan : Trigonometry  Operator=tan
  s : Outport
  tag scope: s_312=global
  wires:
  w/1 -> Demux/1
  Integrator/1 -> Demux1/1, s/1  "s"
  Demux/3 -> Subsystem2/1(In1), Subsystem1/2(In2), Subsystem/1(In1)  "wz"
  Gain/1 -> Subsystem/2(In2)
  Demux/1 -> Gain1/1, Subsystem1/1(In1), Gain/1  "wx"
  Demux1/3 -> Subsystem2/3(In3), Subsystem1/3(In3), Subsystem/3(In3)  "psi"
  Subsystem/1(Out1) -> Divide/1
  Cos/1 -> Divide/2
  Demux1/2 -> Cos/1, Tan/1  "theta"
  Divide/1 -> Mux/1
  Subsystem1/1(Out1) -> Mux/2
  Gain1/1 -> Subsystem2/2(In2)
  Tan/1 -> Product/1
  Subsystem2/1(Out1) -> Product/2
  Product/1 -> Sum/2
  Demux/2 -> Sum/1  "wy"
  Sum/1 -> Mux/3
  Mux/1 -> Integrator/1  "sdot"
  s0/1 -> Integrator/2
  Integrator/State -> [s_312]

== system complete_model_sim_nolib/Kinematics/Kinematics 312/s_312 - A ==
  s : Inport
  Demux : Demux  Outputs=3
  Product : Product  Inputs=3  Multiplication=Matrix(*)
  R1 : Subsystem
  R2 : Subsystem
  R3 : Subsystem
  A : Outport
  wires:
  s/1 -> Demux/1  "s"
  R1/1(R1) -> Product/2
  R3/1(R3) -> Product/3
  R2/1(R2) -> Product/1
  Product/1 -> A/1
  Demux/2 -> R1/1(x)  "theta"
  Demux/1 -> R3/1(x)  "phi"
  Demux/3 -> R2/1(x)  "psi"

== system complete_model_sim_nolib/Kinematics/Kinematics 312/s_313 - A ==
  s : Inport
  Demux : Demux  Outputs=3
  Product : Product  Inputs=3  Multiplication=Matrix(*)
  R1 : Subsystem
  R3_1 : Subsystem
  R3_2 : Subsystem
  A : Outport
  wires:
  Demux/3 -> R3_2/1(x)  "psi"
  Demux/1 -> R3_1/1(x)  "phi"
  Demux/2 -> R1/1(x)  "theta"
  Product/1 -> A/1
  R1/1(R1) -> Product/2
  s/1 -> Demux/1  "s"
  R3_1/1(R3) -> Product/3
  R3_2/1(R3) -> Product/1

== system complete_model_sim_nolib/Kinematics/Kinematics 313/A - s_313 ==
  A : Inport
  Acos : Trigonometry  Operator=acos
  Atan1 : Trigonometry  Operator=atan2
  Atan2 : Trigonometry  Operator=atan2
  Gain : Gain  Gain=-1
  Mux : Mux  Inputs=3
  Selector : Selector  NumberOfDimensions=2  InputPortWidth=3  IndexOptions=Index vector (dialog),Index vector (dialog)  Indices=3,1  OutputSizes=1,1
  Selector1 : Selector  NumberOfDimensions=2  InputPortWidth=3  IndexOptions=Index vector (dialog),Index vector (dialog)  Indices=3,2  OutputSizes=1,1
  Selector2 : Selector  NumberOfDimensions=2  InputPortWidth=3  IndexOptions=Index vector (dialog),Index vector (dialog)  Indices=3,3  OutputSizes=1,1
  Selector3 : Selector  NumberOfDimensions=2  InputPortWidth=3  IndexOptions=Index vector (dialog),Index vector (dialog)  Indices=1,3  OutputSizes=1,1
  Selector4 : Selector  NumberOfDimensions=2  InputPortWidth=3  IndexOptions=Index vector (dialog),Index vector (dialog)  Indices=2,3  OutputSizes=1,1
  s : Outport
  wires:
  Acos/1 -> Mux/2  "theta"
  Selector/1 -> Atan2/1  "a31"
  Selector1/1 -> Gain/1  "a32"
  Selector3/1 -> Atan1/1  "a13"
  Selector2/1 -> Acos/1  "a33"
  A/1 -> Selector4/1, Selector3/1, Selector/1, Selector1/1, Selector2/1
  Atan2/1 -> Mux/1  "phi"
  Atan1/1 -> Mux/3  "psi"
  Gain/1 -> Atan2/2
  Selector4/1 -> Atan1/2  "a23"
  Mux/1 -> s/1

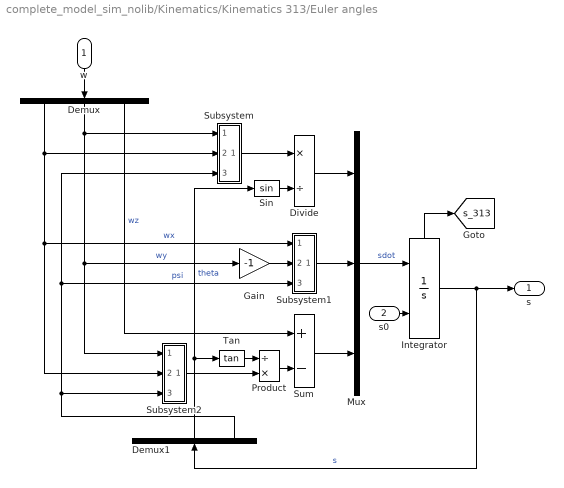
== system complete_model_sim_nolib/Kinematics/Kinematics 313/Euler angles ==
  w : Inport
  s0 : Inport  Port=2
  Demux : Demux  Outputs=3
  Demux1 : Demux  Outputs=3
  Divide : Product  Inputs=*/
  Gain : Gain  Gain=-1
  Integrator : Integrator  InitialConditionSource=external  InitialCondition=s0  WrapState=on  WrappedStateUpperValue=2*pi  WrappedStateLowerValue=0  ShowStatePort=on
  Mux : Mux  Inputs=3
  Product : Product  Inputs=/*
  Sin : Trigonometry
  Subsystem : Subsystem
  Subsystem1 : Subsystem
  Subsystem2 : Subsystem
  Sum : Sum  Inputs=+-
  Tan : Trigonometry  Operator=tan
  s : Outport
  tag scope: s_313=global
  wires:
  Mux/1 -> Integrator/1  "sdot"
  Sum/1 -> Mux/3
  Demux/2 -> Subsystem/1(In1), Subsystem2/1(In1), Gain/1  "wy"
  Product/1 -> Sum/2
  Subsystem2/1(Out1) -> Product/2
  Tan/1 -> Product/1
  Subsystem1/1(Out1) -> Mux/2
  Divide/1 -> Mux/1
  Demux1/2 -> Sin/1, Tan/1  "theta"
  Subsystem/1(Out1) -> Divide/1
  Demux1/3 -> Subsystem/3(In3), Subsystem1/3(In3), Subsystem2/3(In3)  "psi"
  Demux/1 -> Subsystem2/2(In2), Subsystem1/1(In1), Subsystem/2(In2)  "wx"
  Demux/3 -> Sum/1  "wz"
  Integrator/1 -> Demux1/1, s/1  "s"
  w/1 -> Demux/1
  Sin/1 -> Divide/2
  Gain/1 -> Subsystem1/2(In2)
  s0/1 -> Integrator/2
  Integrator/State -> [s_313]

== system complete_model_sim_nolib/Kinematics/Kinematics 313/s_312 - A ==
  s : Inport
  Demux : Demux  Outputs=3
  Product : Product  Inputs=3  Multiplication=Matrix(*)
  R1 : Subsystem
  R2 : Subsystem
  R3 : Subsystem
  A : Outport
  wires:
  s/1 -> Demux/1  "s"
  R1/1(R1) -> Product/2
  R3/1(R3) -> Product/3
  R2/1(R2) -> Product/1
  Product/1 -> A/1
  Demux/2 -> R1/1(x)  "theta"
  Demux/1 -> R3/1(x)  "phi"
  Demux/3 -> R2/1(x)  "psi"

== system complete_model_sim_nolib/Kinematics/Kinematics 313/s_313 - A ==
  s : Inport
  Demux : Demux  Outputs=3
  Product : Product  Inputs=3  Multiplication=Matrix(*)
  R1 : Subsystem
  R3_1 : Subsystem
  R3_2 : Subsystem
  A : Outport
  wires:
  Demux/3 -> R3_2/1(x)  "psi"
  Demux/1 -> R3_1/1(x)  "phi"
  Demux/2 -> R1/1(x)  "theta"
  Product/1 -> A/1
  R1/1(R1) -> Product/2
  s/1 -> Demux/1  "s"
  R3_1/1(R3) -> Product/3
  R3_2/1(R3) -> Product/1

== system complete_model_sim_nolib/Kinematics/System switcher/Compare To Constant ==
  u : Inport
  Compare : RelationalOperator  Operator=<  OutDataTypeStr=boolean
  Constant : Constant  DisableCoverage=on  Value=const  OutDataTypeStr=Inherit: Inherit via back propagation
  y : Outport
  wires:
  u/1 -> Compare/1
  Constant/1 -> Compare/2
  Compare/1 -> y/1

== system complete_model_sim_nolib/Kinematics/System switcher/Compare To Constant1 ==
  u : Inport
  Compare : RelationalOperator  Operator=<  OutDataTypeStr=boolean
  Constant : Constant  DisableCoverage=on  Value=const  OutDataTypeStr=Inherit: Inherit via back propagation
  y : Outport
  wires:
  u/1 -> Compare/1
  Constant/1 -> Compare/2
  Compare/1 -> y/1

== system complete_model_sim_nolib/Sun Sensor/Sun Sensor Modeling/Cross Product ==
  note: Cross product of two 3x1 vectors a=[a1 a2 a3], b=[b1 b2 b3]:
      | y = a x b = (a2b3-a3b2)i + (a3b1-a1b3)j + (a1b2-a2b1)k
  a : Inport
  b : Inport  Port=2
  Element Product : Product  RndMeth=Simplest
  Selector2 : Selector  InputPortWidth=6  IndexOptions=Index vector (dialog)  Indices=[1 2 3]  OutputSizes=1
  Selector3 : Selector  InputPortWidth=6  IndexOptions=Index vector (dialog)  Indices=[4 5 6]  OutputSizes=1
  Sum : Sum  Inputs=+|-  RndMeth=Simplest
  a elements : Selector  InputPortWidth=3  IndexOptions=Index vector (dialog)  Indices=[2 3 1 3 1 2]  OutputSizes=1
  b elements : Selector  InputPortWidth=3  IndexOptions=Index vector (dialog)  Indices=[3 1 2 2 3 1]  OutputSizes=1
  y : Outport
  wires:
  Selector3/1 -> Sum/2
  Selector2/1 -> Sum/1
  Element Product/1 -> Selector2/1, Selector3/1
  b/1 -> b elements/1
  b elements/1 -> Element Product/2
  a elements/1 -> Element Product/1
  Sum/1 -> y/1
  a/1 -> a elements/1

== system complete_model_sim_nolib/Sun Sensor/Sun Sensor Modeling/Normalize Vector ==
  In1 : Inport
  Constant : Constant
  Demux : Demux  Outputs=[-1 1]
  Divide : Product  Inputs=*/  OutDataTypeStr=double
  Ground : Ground
  Math Function : Math  Operator=square  SignedPower=on
  Math Function1 : Math  Operator=sqrt  SignedPower=on
  Mux : Mux  Inputs=2
  Mux1 : Mux  Inputs=2
  Product : Product  RndMeth=Zero
  Sum of Elements : Sum  Inputs=+
  Switch : Switch  Criteria=u2 > Threshold  Threshold=maxzero  SaturateOnIntegerOverflow=off  InputSameDT=off
  Out1 : Outport  VectorParamsAs1DForOutWhenUnconnected=off
  wires:
  Ground/1 -> Product/2
  Product/1 -> Mux1/1
  Constant/1 -> Mux1/2
  Mux1/1 -> Switch/3
  Sum of Elements/1 -> Math Function1/1
  Math Function/1 -> Sum of Elements/1
  Demux/2 -> Divide/2
  Demux/1 -> Divide/1
  Switch/1 -> Demux/1
  Mux/1 -> Switch/1
  Math Function1/1 -> Mux/2, Switch/2
  In1/1 -> Product/1, Math Function/1, Mux/1
  Divide/1 -> Out1/1

== system complete_model_sim_nolib/Sun Sensor/Sun Sensor Modeling/Normalize Vector1 ==
  In1 : Inport
  Constant : Constant
  Demux : Demux  Outputs=[-1 1]
  Divide : Product  Inputs=*/  OutDataTypeStr=double
  Ground : Ground
  Math Function : Math  Operator=square  SignedPower=on
  Math Function1 : Math  Operator=sqrt  SignedPower=on
  Mux : Mux  Inputs=2
  Mux1 : Mux  Inputs=2
  Product : Product  RndMeth=Zero
  Sum of Elements : Sum  Inputs=+
  Switch : Switch  Criteria=u2 > Threshold  Threshold=maxzero  SaturateOnIntegerOverflow=off  InputSameDT=off
  Out1 : Outport  VectorParamsAs1DForOutWhenUnconnected=off
  wires:
  Ground/1 -> Product/2
  Product/1 -> Mux1/1
  Constant/1 -> Mux1/2
  Mux1/1 -> Switch/3
  Sum of Elements/1 -> Math Function1/1
  Math Function/1 -> Sum of Elements/1
  Demux/2 -> Divide/2
  Demux/1 -> Divide/1
  Switch/1 -> Demux/1
  Mux/1 -> Switch/1
  Math Function1/1 -> Mux/2, Switch/2
  In1/1 -> Product/1, Math Function/1, Mux/1
  Divide/1 -> Out1/1

== system complete_model_sim_nolib/Attitude Determination  1/Enabled Subsystem/S/Cross Product ==
  note: Cross product of two 3x1 vectors a=[a1 a2 a3], b=[b1 b2 b3]:
      | y = a x b = (a2b3-a3b2)i + (a3b1-a1b3)j + (a1b2-a2b1)k
  a : Inport
  b : Inport  Port=2
  Element Product : Product  RndMeth=Simplest
  Selector2 : Selector  InputPortWidth=6  IndexOptions=Index vector (dialog)  Indices=[1 2 3]  OutputSizes=1
  Selector3 : Selector  InputPortWidth=6  IndexOptions=Index vector (dialog)  Indices=[4 5 6]  OutputSizes=1
  Sum : Sum  Inputs=+|-  RndMeth=Simplest
  a elements : Selector  InputPortWidth=3  IndexOptions=Index vector (dialog)  Indices=[2 3 1 3 1 2]  OutputSizes=1
  b elements : Selector  InputPortWidth=3  IndexOptions=Index vector (dialog)  Indices=[3 1 2 2 3 1]  OutputSizes=1
  y : Outport
  wires:
  Selector3/1 -> Sum/2
  Selector2/1 -> Sum/1
  Element Product/1 -> Selector2/1, Selector3/1
  b/1 -> b elements/1
  b elements/1 -> Element Product/2
  a elements/1 -> Element Product/1
  Sum/1 -> y/1
  a/1 -> a elements/1

== system complete_model_sim_nolib/Attitude Determination  1/Enabled Subsystem/S/Cross Product1 ==
  note: Cross product of two 3x1 vectors a=[a1 a2 a3], b=[b1 b2 b3]:
      | y = a x b = (a2b3-a3b2)i + (a3b1-a1b3)j + (a1b2-a2b1)k
  a : Inport
  b : Inport  Port=2
  Element Product : Product  RndMeth=Simplest
  Selector2 : Selector  InputPortWidth=6  IndexOptions=Index vector (dialog)  Indices=[1 2 3]  OutputSizes=1
  Selector3 : Selector  InputPortWidth=6  IndexOptions=Index vector (dialog)  Indices=[4 5 6]  OutputSizes=1
  Sum : Sum  Inputs=+|-  RndMeth=Simplest
  a elements : Selector  InputPortWidth=3  IndexOptions=Index vector (dialog)  Indices=[2 3 1 3 1 2]  OutputSizes=1
  b elements : Selector  InputPortWidth=3  IndexOptions=Index vector (dialog)  Indices=[3 1 2 2 3 1]  OutputSizes=1
  y : Outport
  wires:
  Selector3/1 -> Sum/2
  Selector2/1 -> Sum/1
  Element Product/1 -> Selector2/1, Selector3/1
  b/1 -> b elements/1
  b elements/1 -> Element Product/2
  a elements/1 -> Element Product/1
  Sum/1 -> y/1
  a/1 -> a elements/1

== system complete_model_sim_nolib/Attitude Determination  1/Enabled Subsystem/S/Normalize Vector ==
  In1 : Inport
  Constant : Constant
  Demux : Demux  Outputs=[-1 1]
  Divide : Product  Inputs=*/  OutDataTypeStr=double
  Ground : Ground
  Math Function : Math  Operator=square  SignedPower=on
  Math Function1 : Math  Operator=sqrt  SignedPower=on
  Mux : Mux  Inputs=2
  Mux1 : Mux  Inputs=2
  Product : Product  RndMeth=Zero
  Sum of Elements : Sum  Inputs=+
  Switch : Switch  Criteria=u2 > Threshold  Threshold=maxzero  SaturateOnIntegerOverflow=off  InputSameDT=off
  Out1 : Outport  VectorParamsAs1DForOutWhenUnconnected=off
  wires:
  Ground/1 -> Product/2
  Product/1 -> Mux1/1
  Constant/1 -> Mux1/2
  Mux1/1 -> Switch/3
  Sum of Elements/1 -> Math Function1/1
  Math Function/1 -> Sum of Elements/1
  Demux/2 -> Divide/2
  Demux/1 -> Divide/1
  Switch/1 -> Demux/1
  Mux/1 -> Switch/1
  Math Function1/1 -> Mux/2, Switch/2
  In1/1 -> Product/1, Math Function/1, Mux/1
  Divide/1 -> Out1/1

== system complete_model_sim_nolib/Attitude Determination  1/Enabled Subsystem/V/Cross Product ==
  note: Cross product of two 3x1 vectors a=[a1 a2 a3], b=[b1 b2 b3]:
      | y = a x b = (a2b3-a3b2)i + (a3b1-a1b3)j + (a1b2-a2b1)k
  a : Inport
  b : Inport  Port=2
  Element Product : Product  RndMeth=Simplest
  Selector2 : Selector  InputPortWidth=6  IndexOptions=Index vector (dialog)  Indices=[1 2 3]  OutputSizes=1
  Selector3 : Selector  InputPortWidth=6  IndexOptions=Index vector (dialog)  Indices=[4 5 6]  OutputSizes=1
  Sum : Sum  Inputs=+|-  RndMeth=Simplest
  a elements : Selector  InputPortWidth=3  IndexOptions=Index vector (dialog)  Indices=[2 3 1 3 1 2]  OutputSizes=1
  b elements : Selector  InputPortWidth=3  IndexOptions=Index vector (dialog)  Indices=[3 1 2 2 3 1]  OutputSizes=1
  y : Outport
  wires:
  Selector3/1 -> Sum/2
  Selector2/1 -> Sum/1
  Element Product/1 -> Selector2/1, Selector3/1
  b/1 -> b elements/1
  b elements/1 -> Element Product/2
  a elements/1 -> Element Product/1
  Sum/1 -> y/1
  a/1 -> a elements/1
